simulink model "q2"  (R2024a)
settings: Solver=VariableStepAuto  StartTime=0.0  StopTime=10.0  RelTol=1e-3
model workspace (MAT data in the model file):
  B = Simulink.Parameter
  B.Value = 100
  B.Complexity = 'real'
  B.Dimensions = [1 1]
  B.DataType = 'auto'
settings Model: Creator=mvajhi  LastModifiedBy=mvajhi

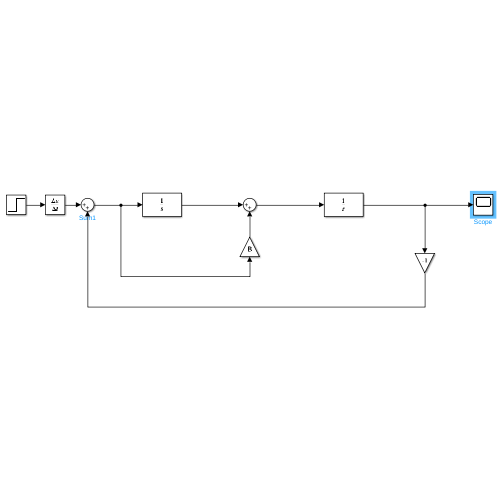
[thumbnail: Simulink's stored preview of the top-level diagram]
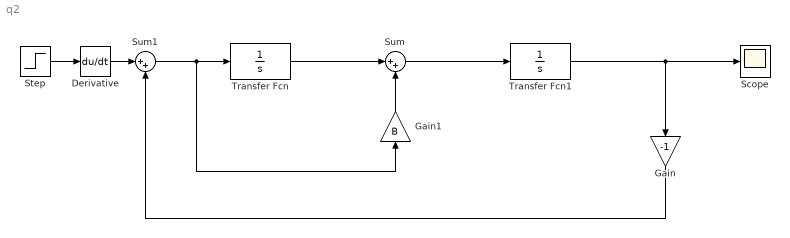
== system q2 ==
  Derivative : Derivative
  Gain : Gain  Gain=-1
  Gain1 : Gain  Gain=B
  Scope : Scope
  Step : Step  Time=0.001  SampleTime=0
  Sum : Sum  Inputs=|++
  Sum1 : Sum  Inputs=|++
  Transfer Fcn : TransferFcn  Denominator=[1 0]
  Transfer Fcn1 : TransferFcn  Denominator=[1 0]
  wires:
  Transfer Fcn1/1 -> Gain/1, Scope/1
  Transfer Fcn/1 -> Sum/1
  Sum/1 -> Transfer Fcn1/1
  Gain1/1 -> Sum/2
  Gain/1 -> Sum1/2
  Sum1/1 -> Gain1/1, Transfer Fcn/1
  Derivative/1 -> Sum1/1
  Step/1 -> Derivative/1
